simulink model "untitled"  (R2023b)
settings: Solver=VariableStepAuto  StartTime=0.0  StopTime=10.0  RelTol=1e-3
settings Model: Creator=akrom  LastModifiedBy=akrom

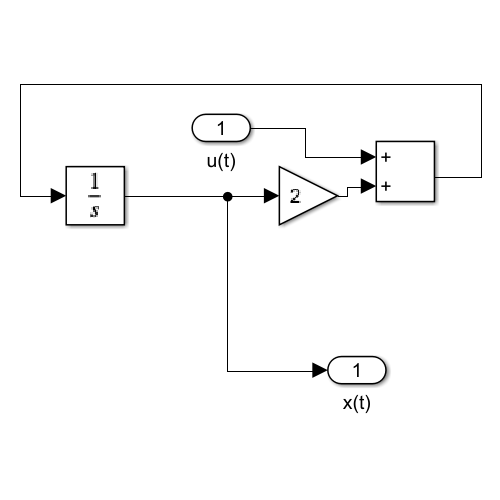
[thumbnail: Simulink's stored preview of the top-level diagram]
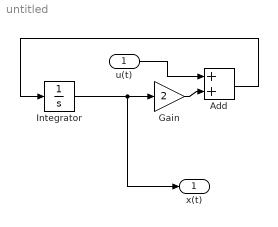
== system untitled ==
  u(t) : Inport
  Add : Sum
  Gain : Gain  Gain=2
  Integrator : Integrator
  x(t) : Outport
  wires:
  Integrator/1 -> Gain/1, x(t)/1
  u(t)/1 -> Add/1
  Add/1 -> Integrator/1
  Gain/1 -> Add/2
